simulink model "SORU1_j"  (R2018b)
settings: Solver=VariableStepAuto  StartTime=0.0  StopTime=100  RelTol=1e-3
settings Model: Creator=Fatih  LastModifiedBy=Fatih

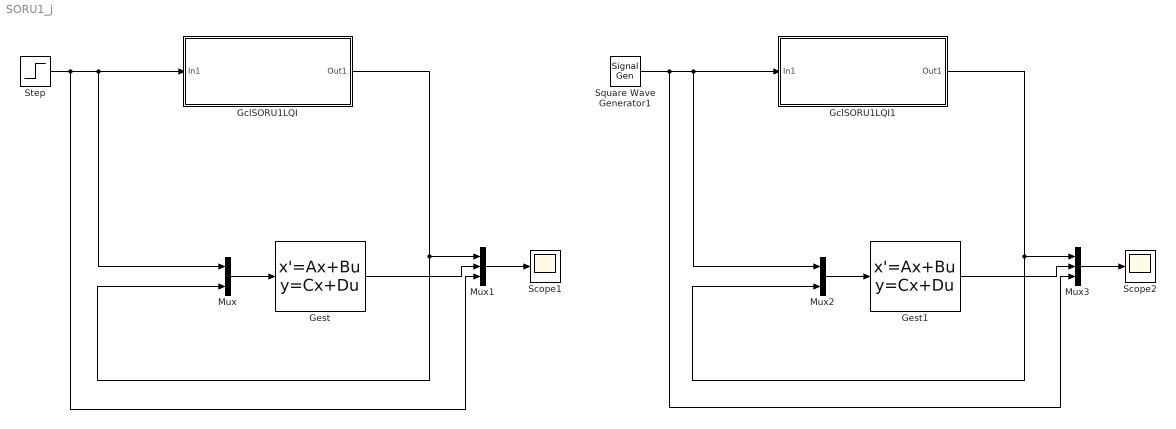
== system SORU1_j ==
  GclSORU1LQI : Subsystem
  GclSORU1LQI1 : Subsystem
  Gest : StateSpace  A=[-0.5 -7.2;0.5 -8.1]  B=[0.5 6.2;0 7.6]  C=[0 1;1 0;0 1]  D=[0 0;0 0;0 0]  InitialCondition=0
  Gest1 : StateSpace  A=[-0.5 -7.2;0.5 -8.1]  B=[0.5 6.2;0 7.6]  C=[0 1;1 0;0 1]  D=[0 0;0 0;0 0]  InitialCondition=0
  Mux : Mux  Inputs=2
  Mux1 : Mux  Inputs=3
  Mux2 : Mux  Inputs=2
  Mux3 : Mux  Inputs=3
  Scope1 : Scope
  Scope2 : Scope
  Square Wave Generator1 : SignalGenerator  WaveForm=square  Units=rad/sec
  Step : Step  SampleTime=0
  wires:
  Mux/1 -> Gest/1
  Mux1/1 -> Scope1/1
  Gest/1 -> Mux1/2
  GclSORU1LQI/1(Out1) -> Mux1/1, Mux/2
  Gest1/1 -> Mux3/2
  GclSORU1LQI1/1(Out1) -> Mux3/1, Mux2/2
  Square Wave Generator1/1 -> Mux3/3, Mux2/1, GclSORU1LQI1/1(In1)
  Mux2/1 -> Gest1/1
  Mux3/1 -> Scope2/1
  Step/1 -> Mux1/3, Mux/1, GclSORU1LQI/1(In1)

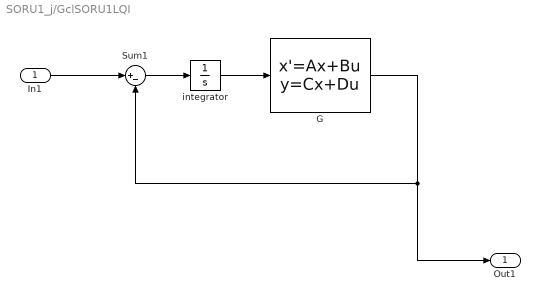
== system SORU1_j/GclSORU1LQI ==
  In1 : Inport
  G : StateSpace  A=[-0.6225 -1.1125;0.5 -0.5]  B=[0.1581;0]  C=[0 1]  D=0  InitialCondition=0
  Sum1 : Sum  Inputs=|+-
  integrator : Integrator
  Out1 : Outport
  wires:
  In1/1 -> Sum1/1
  integrator/1 -> G/1
  Sum1/1 -> integrator/1
  G/1 -> Out1/1, Sum1/2

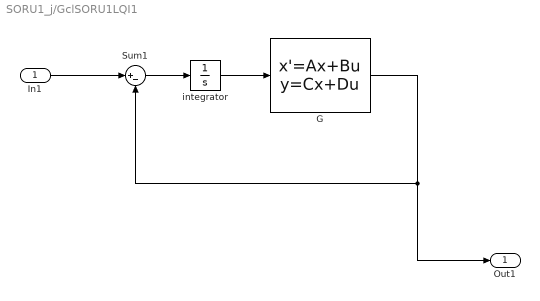
== system SORU1_j/GclSORU1LQI1 ==
  In1 : Inport
  G : StateSpace  A=[-0.6225 -1.1125;0.5 -0.5]  B=[0.1581;0]  C=[0 1]  D=0  InitialCondition=0
  Sum1 : Sum  Inputs=|+-
  integrator : Integrator
  Out1 : Outport
  wires:
  In1/1 -> Sum1/1
  integrator/1 -> G/1
  Sum1/1 -> integrator/1
  G/1 -> Out1/1, Sum1/2
